simulink model "self1"  (R2013b)
settings: Solver=ode45  StartTime=0.0  StopTime=10.0  RelTol=1e-3
libraries: embdlinuxlib x2
settings Model: Creator=mainster  LastModifiedBy=mainster

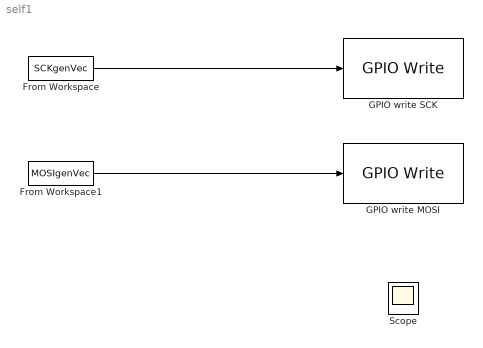
== system self1 ==
  From Workspace : FromWorkspace  VariableName=SCKgenVec  OutDataTypeStr=boolean  SampleTime=0
  From Workspace1 : FromWorkspace  VariableName=MOSIgenVec  OutDataTypeStr=boolean  SampleTime=0
  "GPIO write MOSI " : embdlinuxlib/GPIO Write  board=Model B Rev2  gpio=10  direction=Output  blockPlatform=Raspberry Pi
  GPIO write SCK : embdlinuxlib/GPIO Write  board=Model B Rev2  gpio=11  direction=Output  blockPlatform=Raspberry Pi
  Scope : Scope
  wires:
  From Workspace/1 -> GPIO write SCK/1
  From Workspace1/1 -> "GPIO write MOSI "/1
